simulink model "sampleModel1998"  (R2023a)
settings: Solver=VariableStepAuto  StartTime=0.0  StopTime=10.0  RelTol=1e-3
libraries: hdlsllib x2, simulink x1
settings Model: Creator=user1  LastModifiedBy=user1

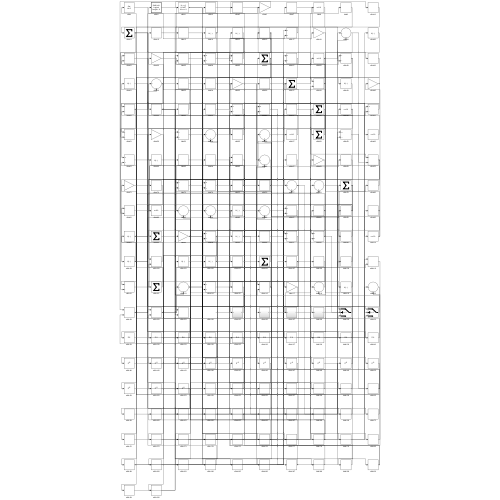
[thumbnail: Simulink's stored preview of the top-level diagram]
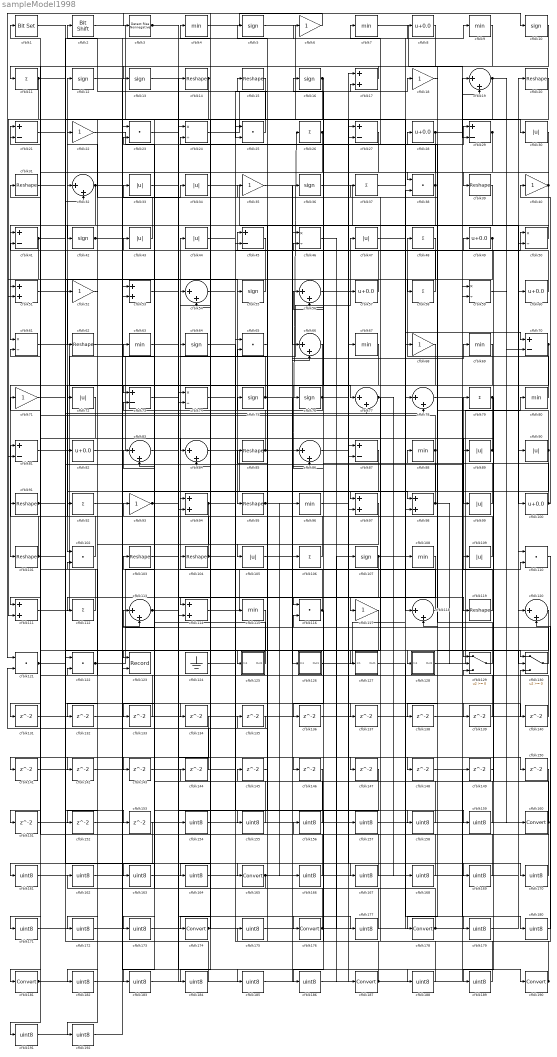
== system sampleModel1998 ==
  cfblk1 : simulink/Logic and Bit Operations/Bit Set  iBit=0
      settings: LibrarySourceBlock=|
      | hdlsllib/Logic and Bit
      | Operations/Bit Set
  cfblk{5,10,12..13,16,36,42,55,64,75..76,107} (12 alike) : Signum
  cfblk{8,28,49,57,60,82,100} (7 alike) : Bias  Bias=0.0  SaturateOnIntegerOverflow=off
  cfblk{14..15,20,31,39,62,85,91,95,101,103..104,119} (13 alike) : Reshape
  cfblk{23,25,38,65,102,110,116,121..122} (9 alike) : DotProduct  OutDataTypeStr=Inherit: Inherit via internal rule
  cfblk{30,33..34,43..44,47,72,89..90,99,105,109} (12 alike) : Abs  SaturateOnIntegerOverflow=off
  cfblk{11,26,37,48,58,79,92,106,112} (9 alike) : Sum  Inputs=+
  cfblk{4,7,9,63,67,69,80,88,96,108,115} (11 alike) : MinMax
  cfblk{17,51,53,94,97..98,111,114} (8 alike) : Sum
  cfblk{19,32,54,56,66,77..78,83..84,86,113,118,120} (13 alike) : Sum  Inputs=|++
  cfblk{6,18,22,35,40,52,68,71,93,117} (10 alike) : Gain
  cfblk123 : Record  FileSettingsInternal="{\"entries\":[{\"content\":{\"excelSettings\":{\"content\":{},\"type\":\"Streamout.ExcelSettings\"}},\"type\":\"Streamout.FileSettingStorage\",\"uuid\":\"\"}],\"packageUris\":[\"http:\\/\\/schema.mathworks.com\\/mf0\\/streamout_blocks\\/R2020a\"],\"version\":\"1.0\"}"  Layout=[1 1]  SignalsInternal="{\"entries\":[{\"content\":{\"signals\":[{\"content\":{\"blockPath\":[],\"dimensions\":[1],\"domain\":\"\",\"lineColor\":\"#a2142f\",\"plots\":[1],\"port\":1,\"signalID\":5757,\"signalName\":\"XY Graph:1\"},\"type\":\"RecordBlkView.Signal\",\"uuid\":\"\"},{\"content\":{\"blockPath\":[],\"dimensions\":[1],\"domain\":\"\",\"lineColor\":\"#139fff\",\"plots\":[1],\"port\":2,\"signalID\":5760,\"signalName\":\"XY Graph:2\"},\"type\":\"RecordBlkView.Signal\",\"uuid\":\"\"}]},\"type\":\"RecordBlkView.InputSignals\",\"uuid\":\"\"}],\"packageUris\":[\"http:\\/\\/schema.mathworks.com\\/mf0\\/streamout_blocks\\/R2020a\"],\"version\":\"1.0\"}"  VisualizationBindings="{\"xyplotplugin\":{\"info\":[{\"series\":[{\"bindingParametersList\":[{\"parameter\":\"X-Axis\",\"signalID\":5757,\"signalName\":\"XY Graph:1\"},{\"parameter\":\"Y-Axis\",\"signalID\":5760,\"signalName\":\"XY Graph:2\"}],\"seriesID\":6724}],\"subplotID\":1}]}}"  CompatibilityTag=XY  st=-1
  cfblk124 : Ground
  cfblk125 : Subsystem
      settings: LibrarySourceBlock=|
      | hdlsllib/Ports &
      | Subsystems/Subsystem
  cfblk126 : Subsystem
      settings: LibrarySourceBlock=|
      | hdlsllib/Ports &
      | Subsystems/Subsystem
  cfblk127 : Subsystem
      settings: LibrarySourceBlock=|
      | hdlsllib/Ports &
      | Subsystems/Subsystem
  cfblk128 : Subsystem
      settings: LibrarySourceBlock=|
      | hdlsllib/Ports &
      | Subsystems/Subsystem
  cfblk129 : Switch  SaturateOnIntegerOverflow=off  InputSameDT=off
  cfblk130 : Switch  SaturateOnIntegerOverflow=off  InputSameDT=off
  cfblk{131..153} (23 alike) : Delay  SampleTime=1
  cfblk{154..159,161..164,166..173,175,177,179..180,182..186,188..189,191..192} (31 alike) : DataTypeConversion  OutDataTypeStr=uint8  SaturateOnIntegerOverflow=off  RndMeth=Floor
  cfblk{160,165,174,176,178,181,187,190} (8 alike) : DataTypeConversion  SaturateOnIntegerOverflow=off  RndMeth=Floor
  cfblk2 : hdlsllib/Logic and Bit Operations/Bit Shift  mode=Shift Left Logical  N=0
  cfblk{21,27,29,41,45,70,73,81,87} (9 alike) : Sum  Inputs=+-
  cfblk{24,46,50,59,61,74} (6 alike) : Product  Inputs=*/  RndMeth=Zero  SaturateOnIntegerOverflow=on
  cfblk3 : hdlsllib/Logic and Bit Operations/Detect Rise Nonnegative  vinit=0  OutDataTypeStr=boolean
  wires:
  cfblk106/1 -> cfblk12/1
  cfblk61/1 -> cfblk77/1
  cfblk104/1 -> cfblk44/1, cfblk119/1
  cfblk80/1 -> cfblk48/1
  cfblk125/1(Out1) -> cfblk93/1
  cfblk85/1 -> cfblk26/1, cfblk54/1
  cfblk32/1 -> cfblk61/1, cfblk6/1
  cfblk60/1 -> cfblk32/1
  cfblk3/1 -> cfblk150/1, cfblk158/1
  cfblk98/1 -> cfblk33/1, cfblk129/2
  cfblk45/1 -> cfblk62/1
  cfblk128/1(Out1) -> cfblk80/1
  cfblk48/1 -> cfblk95/1
  cfblk81/1 -> cfblk47/1
  cfblk94/1 -> cfblk117/1, cfblk132/1
  cfblk14/1 -> cfblk121/1, cfblk72/1
  cfblk67/1 -> cfblk101/1
  cfblk57/1 -> cfblk43/1
  cfblk50/1 -> cfblk41/1
  cfblk19/1 -> cfblk42/1, cfblk70/2
  cfblk111/1 -> cfblk23/1
  cfblk58/1 -> cfblk45/1
  cfblk44/1 -> cfblk29/1
  cfblk22/1 -> cfblk28/1
  cfblk118/1 -> cfblk94/1
  cfblk100/1 -> cfblk75/1, cfblk40/1
  cfblk59/1 -> cfblk160/1
  cfblk39/1 -> cfblk125/1(In1)
  cfblk24/1 -> cfblk18/1
  cfblk75/1 -> cfblk96/1, cfblk4/1
  cfblk27/1 -> cfblk181/1
  cfblk2/1 -> cfblk118/1
  cfblk38/1 -> cfblk7/1, cfblk143/1
  cfblk119/1 -> cfblk79/1
  cfblk71/1 -> cfblk165/1
  cfblk63/1 -> cfblk176/1
  cfblk105/1 -> cfblk69/1
  cfblk90/1 -> cfblk102/1, cfblk35/1
  cfblk96/1 -> cfblk17/1
  cfblk53/1 -> cfblk190/1
  cfblk4/1 -> cfblk10/1
  cfblk25/1 -> cfblk2/1
  cfblk18/1 -> cfblk58/1
  cfblk35/1 -> cfblk66/1
  cfblk20/1 -> cfblk38/1
  cfblk126/1(Out1) -> cfblk68/1
  cfblk9/1 -> cfblk13/1
  cfblk77/1 -> cfblk127/1(In1), cfblk168/1
  cfblk79/1 -> cfblk99/1, cfblk189/1
  cfblk82/1 -> cfblk14/1
  cfblk37/1 -> cfblk9/1
  cfblk113/1 -> cfblk146/1, cfblk147/1
  cfblk5/1 -> cfblk57/1
  cfblk55/1 -> cfblk51/1
  cfblk102/1 -> cfblk81/1
  cfblk41/1 -> cfblk32/2, cfblk81/2
  cfblk42/1 -> cfblk97/1, cfblk113/2, cfblk188/1
  cfblk7/1 -> cfblk29/2
  cfblk54/1 -> cfblk25/1
  cfblk101/1 -> cfblk89/1, cfblk123/1, cfblk91/1
  cfblk99/1 -> cfblk88/1
  cfblk109/1 -> cfblk23/2
  cfblk91/1 -> cfblk78/2, cfblk153/1
  cfblk13/1 -> cfblk116/1
  cfblk11/1 -> cfblk25/2, cfblk51/2, cfblk137/1
  cfblk29/1 -> cfblk118/2, cfblk94/2
  cfblk72/1 -> cfblk111/1
  cfblk107/1 -> cfblk78/1, cfblk164/1
  cfblk78/1 -> cfblk130/1
  cfblk34/1 -> cfblk100/1
  cfblk74/1 -> cfblk50/1
  cfblk121/1 -> cfblk52/1, cfblk8/1
  cfblk103/1 -> cfblk110/2
  cfblk92/1 -> cfblk34/1
  cfblk88/1 -> cfblk21/2, cfblk133/1
  cfblk1/1 -> cfblk128/1(In1)
  cfblk66/1 -> cfblk105/1
  cfblk16/1 -> cfblk76/1, cfblk111/2, cfblk173/1
  cfblk122/1 -> cfblk67/1, cfblk66/2
  cfblk46/1 -> cfblk187/1
  cfblk124/1 -> cfblk17/2
  cfblk84/1 -> cfblk126/1(In1)
  cfblk17/1 -> cfblk11/1
  cfblk73/1 -> cfblk130/2
  cfblk93/1 -> cfblk139/1, cfblk140/1
  cfblk47/1 -> cfblk70/1
  cfblk15/1 -> cfblk174/1
  cfblk70/1 -> cfblk92/1, cfblk123/2
  cfblk95/1 -> cfblk98/1, cfblk166/1
  cfblk89/1 -> cfblk82/1, cfblk84/1
  cfblk130/1 -> cfblk116/2
  cfblk49/1 -> cfblk41/2, cfblk54/2
  cfblk36/1 -> cfblk60/1
  cfblk26/1 -> cfblk114/1, cfblk84/2
  cfblk28/1 -> cfblk30/1, cfblk112/1
  cfblk40/1 -> cfblk39/1, cfblk141/1
  cfblk6/1 -> cfblk3/1
  cfblk120/1 -> cfblk178/1
  cfblk112/1 -> cfblk21/1
  cfblk129/1 -> cfblk24/2
  cfblk43/1 -> cfblk22/1
  cfblk76/1 -> cfblk73/1, cfblk73/2, cfblk148/1
  cfblk12/1 -> cfblk129/1
  cfblk116/1 -> cfblk64/1, cfblk136/1
  cfblk21/1 -> cfblk55/1
  cfblk114/1 -> cfblk19/2
  cfblk117/1 -> cfblk131/1
  cfblk131/1 -> cfblk97/2
  cfblk132/1 -> cfblk77/2
  cfblk133/1 -> cfblk122/2
  cfblk51/1 -> cfblk134/1
  cfblk135/1 -> cfblk121/2
  cfblk136/1 -> cfblk130/3
  cfblk137/1 -> cfblk50/2
  cfblk10/1 -> cfblk138/1
  cfblk138/1 -> cfblk19/1
  cfblk139/1 -> cfblk102/2
  cfblk140/1 -> cfblk1/1
  cfblk141/1 -> cfblk114/2
  cfblk69/1 -> cfblk142/1
  cfblk142/1 -> cfblk45/2
  cfblk143/1 -> cfblk74/2
  cfblk144/1 -> cfblk61/2
  cfblk145/1 -> cfblk65/2
  cfblk149/1 -> cfblk129/3
  cfblk30/1 -> cfblk151/1
  cfblk151/1 -> cfblk24/1
  cfblk68/1 -> cfblk152/1
  cfblk152/1 -> cfblk98/2
  cfblk83/1 -> cfblk154/1
  cfblk154/1 -> cfblk106/1
  cfblk65/1 -> cfblk155/1
  cfblk155/1 -> cfblk83/1
  cfblk150/1 -> cfblk156/1
  cfblk156/1 -> cfblk83/2
  cfblk56/1 -> cfblk157/1
  cfblk157/1 -> cfblk90/1
  cfblk158/1 -> cfblk56/1
  cfblk64/1 -> cfblk159/1
  cfblk159/1 -> cfblk56/2
  cfblk160/1 -> cfblk5/1, cfblk49/1
  cfblk8/1 -> cfblk161/1
  cfblk161/1 -> cfblk59/1
  cfblk162/1 -> cfblk59/2
  cfblk115/1 -> cfblk163/1
  cfblk163/1 -> cfblk103/1
  cfblk164/1 -> cfblk115/1
  cfblk165/1 -> cfblk162/1, cfblk110/1
  cfblk166/1 -> cfblk71/1
  cfblk31/1 -> cfblk167/1
  cfblk167/1 -> cfblk104/1
  cfblk168/1 -> cfblk31/1
  cfblk86/1 -> cfblk169/1
  cfblk169/1 -> cfblk85/1
  cfblk33/1 -> cfblk170/1
  cfblk170/1 -> cfblk86/1
  cfblk134/1 -> cfblk171/1
  cfblk171/1 -> cfblk86/2
  cfblk108/1 -> cfblk172/1
  cfblk172/1 -> cfblk20/1
  cfblk173/1 -> cfblk108/1
  cfblk174/1 -> cfblk144/1, cfblk38/2
  cfblk110/1 -> cfblk175/1
  cfblk175/1 -> cfblk15/1
  cfblk176/1 -> cfblk135/1, cfblk107/1
  cfblk23/1 -> cfblk177/1
  cfblk177/1 -> cfblk63/1
  cfblk178/1 -> cfblk149/1, cfblk16/1, cfblk113/1
  cfblk127/1(Out1) -> cfblk179/1
  cfblk179/1 -> cfblk120/1
  cfblk148/1 -> cfblk180/1
  cfblk180/1 -> cfblk120/2
  cfblk181/1 -> cfblk36/1, cfblk74/1
  cfblk52/1 -> cfblk182/1
  cfblk182/1 -> cfblk27/1
  cfblk146/1 -> cfblk183/1
  cfblk183/1 -> cfblk27/2
  cfblk87/1 -> cfblk184/1
  cfblk184/1 -> cfblk122/1
  cfblk62/1 -> cfblk185/1
  cfblk185/1 -> cfblk87/1
  cfblk147/1 -> cfblk186/1
  cfblk186/1 -> cfblk87/2
  cfblk187/1 -> cfblk145/1, cfblk109/1
  cfblk188/1 -> cfblk46/1
  cfblk189/1 -> cfblk46/2
  cfblk190/1 -> cfblk37/1, cfblk65/1
  cfblk153/1 -> cfblk191/1
  cfblk191/1 -> cfblk53/1
  cfblk97/1 -> cfblk192/1
  cfblk192/1 -> cfblk53/2

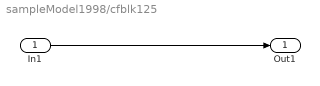
== system sampleModel1998/cfblk125 ==
  In1 : Inport
  Out1 : Outport
  wires:
  In1/1 -> Out1/1

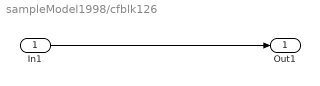
== system sampleModel1998/cfblk126 ==
  In1 : Inport
  Out1 : Outport
  wires:
  In1/1 -> Out1/1

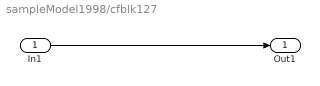
== system sampleModel1998/cfblk127 ==
  In1 : Inport
  Out1 : Outport
  wires:
  In1/1 -> Out1/1

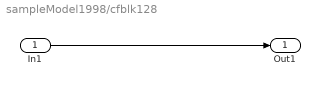
== system sampleModel1998/cfblk128 ==
  In1 : Inport
  Out1 : Outport
  wires:
  In1/1 -> Out1/1
